simulink model "update_entry_model_tester"  (R2020b)
settings: Solver=FixedStepDiscrete  StartTime=0.0  StopTime=81  FixedStep=0.1  RelTol=1e-3
undefined symbols (not defined in the file): DiscIntNeverNeededParam, test_input
libraries: simulink x5
settings Model: Creator=rsub  LastModifiedBy=rsub

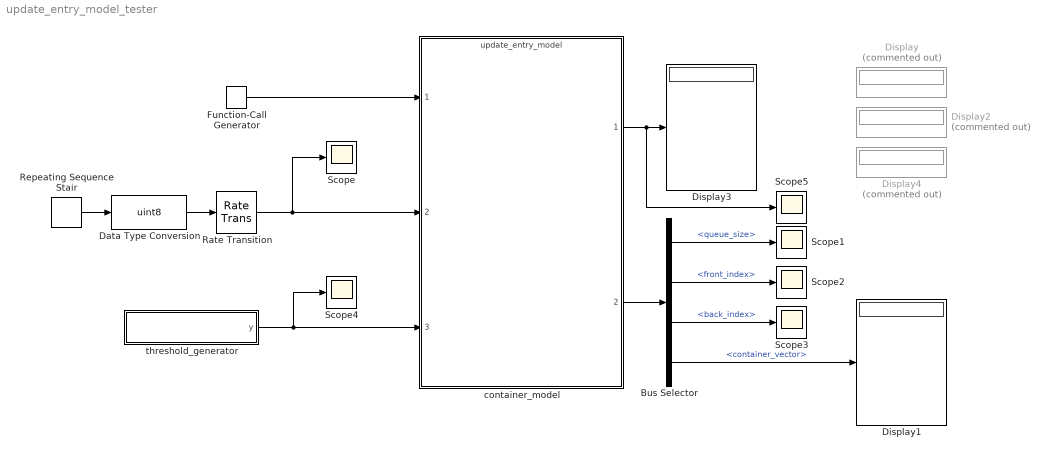
== system update_entry_model_tester ==
  Bus Selector : BusSelector  OutputSignals=queue_size,front_index,back_index,container_vector
  Data Type Conversion : DataTypeConversion  OutDataTypeStr=uint8
  Display : Display  Commented=on
  Display1 : Display
  Display2 : Display  Commented=on
  Display3 : Display
  Display4 : Display  Commented=on
  Function-Call Generator : simulink/Ports & Subsystems/Function-Call Generator  sample_time=5  numberOfIterations=1  DisallowWideOutput=off
  Rate Transition : RateTransition  Integrity=off  Deterministic=off  OutPortSampleTime=5
  Repeating Sequence Stair : simulink/Sources/Repeating Sequence Stair  OutValues=[10:1000].'  tsamp=5  OutMin=[]  OutMax=[]  OutDataTypeStr=double  OutputDataTypeScalingMode=double  OutDataType=fixdt(0,8)  ConRadixGroup=Best Precision: Vector-wise  OutScaling=2^-12
  Scope{,1..5} (6 alike) : Scope
  container_model : ModelReference  ModelNameDialog=update_entry_model.slx  ScheduleRates=on  ModelReferenceVersion=1.592
  threshold_generator : Subsystem
  wires:
  Rate Transition/1 -> Scope/1, container_model/2
  Repeating Sequence Stair/1 -> Data Type Conversion/1
  Data Type Conversion/1 -> Rate Transition/1
  container_model/1 -> Scope5/1, Display3/1
  Function-Call Generator/1 -> container_model/1
  container_model/2 -> Bus Selector/1
  Bus Selector/1 -> Scope1/1  "<queue_size>"
  Bus Selector/2 -> Scope2/1  "<front_index>"
  Bus Selector/3 -> Scope3/1  "<back_index>"
  Bus Selector/4 -> Display1/1  "<container_vector>"
  threshold_generator/1(y) -> Scope4/1, container_model/3

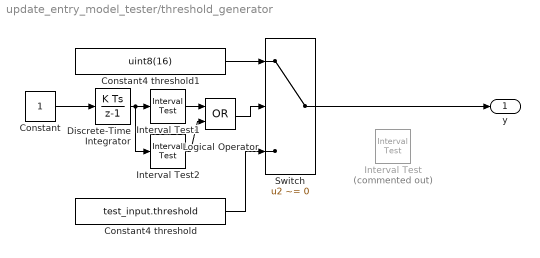
== system update_entry_model_tester/threshold_generator ==
  Constant : Constant
  Constant4 threshold : Constant  Value=test_input.threshold
  Constant4 threshold1 : Constant  Value=uint8(16)
  Discrete-Time Integrator : DiscreteIntegrator  SampleTime=-1  ICPrevOutput=DiscIntNeverNeededParam  ICPrevScaledInput=DiscIntNeverNeededParam
  Interval Test : simulink/Logic and Bit Operations/Interval Test  Commented=on  IntervalClosedRight=on  uplimit=6  IntervalClosedLeft=on  lowlimit=4  OutDataTypeStr=boolean
  Interval Test1 : simulink/Logic and Bit Operations/Interval Test  IntervalClosedRight=on  uplimit=31  IntervalClosedLeft=on  lowlimit=27  OutDataTypeStr=boolean
  Interval Test2 : simulink/Logic and Bit Operations/Interval Test  IntervalClosedRight=on  uplimit=61  IntervalClosedLeft=on  lowlimit=57  OutDataTypeStr=boolean
  Logical Operator : Logic  Operator=OR  AllPortsSameDT=off  OutDataTypeStr=boolean
  Switch : Switch  Criteria=u2 ~= 0
  y : Outport
  wires:
  Constant/1 -> Discrete-Time Integrator/1
  Constant4 threshold1/1 -> Switch/1
  Discrete-Time Integrator/1 -> Interval Test2/1, Interval Test1/1
  Switch/1 -> y/1
  Constant4 threshold/1 -> Switch/3
  Interval Test1/1 -> Logical Operator/1
  Interval Test2/1 -> Logical Operator/2
  Logical Operator/1 -> Switch/2
